simulink model "QAM16_PLL_Model"  (R2019a)
settings: Solver=FixedStepDiscrete  StartTime=0.0  StopTime=inf  FixedStep=1  RelTol=1e-3
undefined symbols (not defined in the file): DiscIntNeverNeededParam, i, jsin
libraries: commdigbbndam3 x3, commchan3 x1, commrandsrc3 x1
settings Model: Creator=vovan  LastModifiedBy=vovan
settings OptimizationCC: BlockReduction=off  DefaultParameterBehavior=Inlined  OptimizeBlockIOStorage=off  BufferReuse=off  GlobalBufferReuse=off  ExpressionFolding=off  PassReuseOutputArgsAs=Individual arguments  LocalBlockOutputs=off  OptimizeBlockOrder=speed  OptimizeDataStoreBuffers=off  BusAssignmentInplaceUpdate=off
settings DebuggingCC: ParameterTunabilityLossMsg=error
settings HardwareCC: TargetBitPerPointer=64  TargetBitPerSizeT=64  TargetBitPerPtrDiffT=64  TargetLongLongMode=on  TargetIntDivRoundTo=Zero  TargetEndianess=LittleEndian  TargetWordSize=64  TargetHWDeviceType=Generic->Custom  ProdEqTarget=off
settings SFSimCC: MATLABDynamicMemAlloc=off
settings RTWCC: SystemTargetFile=systemverilog_dpi_ert.tlc  TemplateMakefile=systemverilog_dpi_ert_default_tmf  Description=SystemVerilog DPI Component Generator  GenerateReport=on  IncludeHyperlinkInReport=on  LaunchReport=on  GenerateTraceInfo=on  GenerateTraceReport=on  GenerateTraceReportSl=on  GenerateTraceReportSf=on  GenerateTraceReportEml=on
settings CodeAppCC: ForceParamTrailComments=on  IgnoreCustomStorageClasses=off  MaxIdLength=256  OperatorAnnotations=on  SimulinkDataObjDesc=on  SFDataObjDesc=on  InsertBlockDesc=on
settings DPIERTTargetCC: TargetFcnLib=ansi_tfl_table_tmw.mat  GenFloatMathFcnCalls=NOT IN USE  TargetLangStandard=C89/C90 (ANSI)  CodeReplacementLibrary=None  UtilityFuncGeneration=Auto  MultiwordTypeDef=System defined  MultiwordLength=2048  DynamicStringBufferSize=256  GenerateFullHeader=on  InferredTypesCompatibility=off  GenerateSampleERTMain=off  GenerateTestInterfaces=off  ModelReferenceCompliant=on  ParMdlRefBuildCompliant=on  CompOptLevelCompliant=off  ConcurrentExecutionCompliant=off  IncludeMdlTerminateFcn=on  GeneratePreprocessorConditionals=Use local settings  CombineOutputUpdateFcns=off  CombineSignalStateStructs=on  GroupInternalDataByFunction=off  SuppressErrorStatus=off  IncludeFileDelimiter=Auto  ERTCustomFileBanners=on  SupportAbsoluteTime=on  LogVarNameModifier=rt_  MatFileLogging=off  MultiInstanceERTCode=on  CodeInterfacePackaging=Reusable function  PurelyIntegerCode=off  SupportNonFinite=on  SupportComplex=on  SupportContinuousTime=on  SupportNonInlinedSFcns=on  RemoveDisableFunc=off  RemoveResetFunc=on  SupportVariableSizeSignals=off  ParenthesesLevel=Nominal  CastingMode=Nominal  PreserveStateflowLocalDataDimensions=off  MATLABClassNameForMDSCustomization=Simulink.SoftwareTarget.TargetSpecificTriggerConfigurationBase  ModelStepFunctionPrototypeControlCompliant=on  CPPClassGenCompliant=off  AutosarCompliant=off  MDXCompliant=off  GRTInterface=off  GenerateAllocFcn=on  UseToolchainInfoCompliant=on  GenerateSharedConstants=on  CoderGroups=[]  AccessMethods=[]  LookupTableObjectStructAxisOrder=1,2,3,4,...  LUTObjectStructOrderExplicitValues=Size,Breakpoints,Table  LUTObjectStructOrderEvenSpacing=Size,Breakpoints,Table  ArrayLayout=Column-major  UnsupportedSFcnMsg=error  ERTHeaderFileRootName=$R$E  ERTSourceFileRootName=$R$E  ERTDataFileRootName=$R_data  GenerateASAP2=off  DSAsUniqueAccess=off  ExtMode=off  ExtModeTransport=0  ExtModeStaticAlloc=off  ExtModeStaticAllocSize=1000000  ExtModeTesting=off  ExtModeMexFile=ext_comm  ExtModeIntrfLevel=Level1  InlinedParameterPlacement=NonHierarchical  TargetOS=BareBoardExample  MultiInstanceErrorCode=Error  RootIOFormat=Part of model data structure  RTWCAPISignals=on  RTWCAPIParams=off  RTWCAPIStates=off  RTWCAPIRootIO=off  ERTSrcFileBannerTemplate=ert_code_template.cgt  ERTHdrFileBannerTemplate=ert_code_template.cgt  ERTDataSrcFileTemplate=ert_code_template.cgt  ERTDataHdrFileTemplate=ert_code_template.cgt  ERTCustomFileTemplate=example_file_process.tlc  EnableDataOwnership=off  SignalDisplayLevel=10  ParamTuneLevel=10  GlobalDataDefinition=Auto  DataDefinitionFile=global.c  GlobalDataReference=Auto  ERTFilePackagingFormat=Modular  RateTransitionBlockCode=Inline  DataReferenceFile=global.h  PreserveExpressionOrder=off  PreserveIfCondition=off  ConvertIfToSwitch=on  PreserveExternInFcnDecls=on  PreserveStaticInFcnDecls=on  SuppressUnreachableDefaultCases=on  EnableSignedLeftShifts=on  EnableSignedRightShifts=on  IndentStyle=K&R  IndentSize=2  NewlineStyle=Default  MaxLineWidth=80  EnableUserReplacementTypes=off  MaxIdInt64=MAX_int64_T  MinIdInt64=MIN_int64_T  MaxIdUint64=MAX_uint64_T  MaxIdInt32=MAX_int32_T  MinIdInt32=MIN_int32_T  MaxIdUint32=MAX_uint32_T  MaxIdInt16=MAX_int16_T  MinIdInt16=MIN_int16_T  MaxIdUint16=MAX_uint16_T  MaxIdInt8=MAX_int8_T  MinIdInt8=MIN_int8_T  MaxIdUint8=MAX_uint8_T  BooleanTrueId=true  BooleanFalseId=false  MemSecPackage=--- None ---  MemSecDataConstants=Default  MemSecDataIO=Default  MemSecDataInternal=Default  MemSecDataParameters=Default  MemSecFuncInitTerm=Default  MemSecFuncExecute=Default  MemSecFuncSharedUtil=Default  GroupConstants=Default  GroupRootInputs=Default  GroupRootOutputs=Default  GroupInternal=Default  GroupParameters=Default  GroupDataTransfer=Default  GroupSharedLocalDataStores=Default  GroupInstanceSpecificParameters=Default  GroupModelData=Default  DPICustomizeSystemVerilogCode=on  DPISystemVerilogTemplate=hdlverifier_dpitb_template.vgt  DPIGenerateTestBench=off  DPITestPointAccessFcnInterface=None  DPIFixedPointDataType=CompatibleCType  DPIPortConnection=Port list  DPICompositeDataType=Flattened

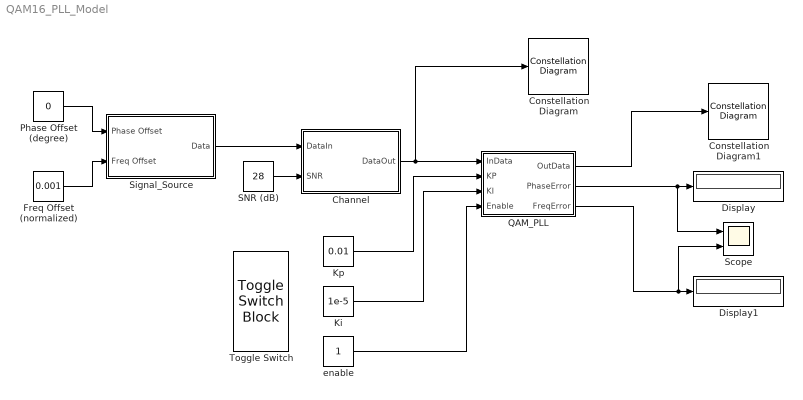
== system QAM16_PLL_Model ==
  Channel : Subsystem
  Constellation Diagram : ConstellationDiagram
  Constellation Diagram1 : ConstellationDiagram
  Display : Display
  Display1 : Display
  Freq Offset (normalized) : Constant  Value=0.001  SampleTime=1
  Ki : Constant  Value=1e-5  SampleTime=1
  Kp : Constant  Value=0.01  SampleTime=1
  Phase Offset (degree) : Constant  Value=0  SampleTime=1
  QAM_PLL : Subsystem
  SNR (dB) : Constant  Value=28  SampleTime=1
  Scope : Scope  NumInputPorts=2
  Signal_Source : Subsystem
  Toggle Switch : ToggleSwitchBlock
      settings: Values={{'Off', 'On'}, [0 1]}
  "enable " : Constant  OutDataTypeStr=boolean  SampleTime=1
  wires:
  Phase Offset (degree)/1 -> Signal_Source/1("Phase Offset ")
  Freq Offset (normalized)/1 -> Signal_Source/2(Freq Offset)
  Signal_Source/1(Data) -> Channel/1(DataIn)
  SNR (dB)/1 -> Channel/2(SNR)
  Channel/1(DataOut) -> QAM_PLL/1(InData), Constellation Diagram/1
  Kp/1 -> QAM_PLL/2(KP)
  Ki/1 -> QAM_PLL/3(KI)
  "enable "/1 -> QAM_PLL/4(Enable)
  QAM_PLL/1(OutData) -> Constellation Diagram1/1
  QAM_PLL/2(PhaseError) -> Scope/1, Display/1
  QAM_PLL/3(FreqError) -> Scope/2, Display1/1

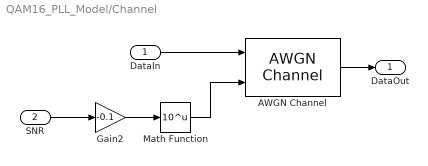
== system QAM16_PLL_Model/Channel ==
  DataIn : Inport
  SNR : Inport  Port=2
  AWGN Channel : commchan3/AWGN Channel  InputProcessing=Columns as channels (frame based)  seed=randseed  noiseMode=Variance from port  EbNodB=10  EsNodB=10  SNRdB=10  bitsPerSym=1  Ps=1  Tsym=1  variance=1
      settings: SourceProductName=Communications Toolbox
  Gain2 : Gain  Gain=-0.1
  Math Function : Math  Operator=10^u  SaturateOnIntegerOverflow=on
  DataOut : Outport
  wires:
  Math Function/1 -> AWGN Channel/2
  Gain2/1 -> Math Function/1
  DataIn/1 -> AWGN Channel/1
  AWGN Channel/1 -> DataOut/1
  SNR/1 -> Gain2/1

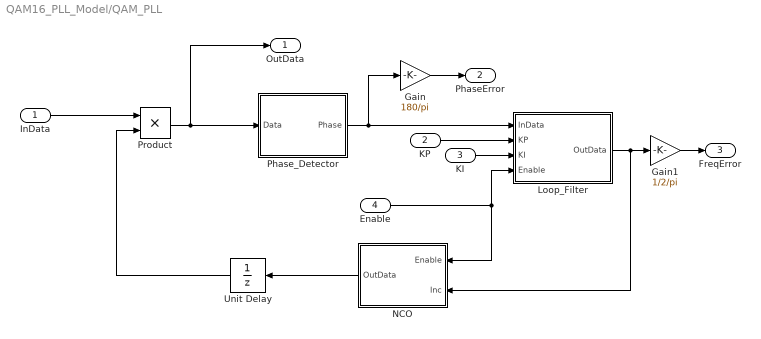
== system QAM16_PLL_Model/QAM_PLL ==
  InData : Inport
  KP : Inport  Port=2
  KI : Inport  Port=3
  Enable : Inport  Port=4
  Gain : Gain  Gain=180/pi
  Gain1 : Gain  Gain=1/2/pi
  Loop_Filter : Subsystem
  NCO : Subsystem
  Phase_Detector : Subsystem
  Product : Product
  Unit Delay : UnitDelay  SampleTime=-1  HasFrameUpgradeWarning=on
  OutData : Outport
  PhaseError : Outport  Port=2
  FreqError : Outport  Port=3
  wires:
  KP/1 -> Loop_Filter/2(KP)
  Enable/1 -> Loop_Filter/4(Enable), NCO/1(Enable)
  Phase_Detector/1(Phase) -> Gain/1, Loop_Filter/1(InData)
  Product/1 -> Phase_Detector/1(Data), OutData/1
  KI/1 -> Loop_Filter/3(KI)
  Loop_Filter/1(OutData) -> Gain1/1, NCO/2(Inc)
  NCO/1(OutData) -> Unit Delay/1
  Unit Delay/1 -> Product/2
  InData/1 -> Product/1
  Gain/1 -> PhaseError/1
  Gain1/1 -> FreqError/1

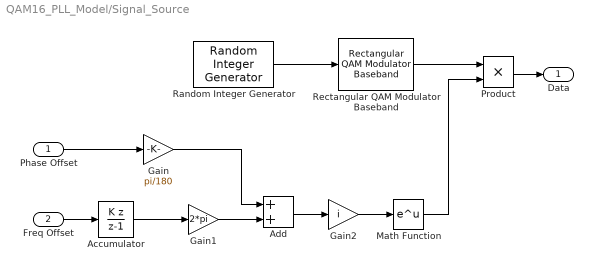
== system QAM16_PLL_Model/Signal_Source ==
  "Phase Offset " : Inport
  Freq Offset : Inport  Port=2
  Accumulator : DiscreteIntegrator  IntegratorMethod=Accumulation: Backward Euler  SampleTime=-1  ICPrevOutput=DiscIntNeverNeededParam  ICPrevScaledInput=DiscIntNeverNeededParam
  Add : Sum
  Gain : Gain  Gain=pi/180
  Gain1 : Gain  Gain=2*pi
  Gain2 : Gain  Gain=i
  Math Function : Math  SaturateOnIntegerOverflow=on
  Product : Product
  Random Integer Generator : commrandsrc3/Random Integer Generator  SetSize=16  SeedSource=Auto  Seed=0  SampleTime=1  SamplesPerFrame=1  OutputDataType=double  SimulateUsing=Interpreted execution
      settings: SourceProductName=Communications Toolbox
  Rectangular QAM Modulator Baseband : commdigbbndam3/Rectangular QAM Modulator Baseband  M=16  InType=Integer  Enc=Gray  Mapping=[0:15]  PowType=Average Power  MinDist=2  AvgPow=1  PeakPow=1  Ph=0  outDtype=double  outWordLen=16  outUDDataType=sfix(16)  outFracLenMode=Best precision  outFracLen=15  outDataTypeStr=double  outLastDataTypeStr=double
      settings: SourceProductName=Communications Toolbox
  Data : Outport
  wires:
  Gain/1 -> Add/1
  Rectangular QAM Modulator Baseband/1 -> Product/1
  Random Integer Generator/1 -> Rectangular QAM Modulator Baseband/1
  Freq Offset/1 -> Accumulator/1
  Gain1/1 -> Add/2
  Add/1 -> Gain2/1
  Gain2/1 -> Math Function/1
  Math Function/1 -> Product/2
  Accumulator/1 -> Gain1/1
  "Phase Offset "/1 -> Gain/1
  Product/1 -> Data/1

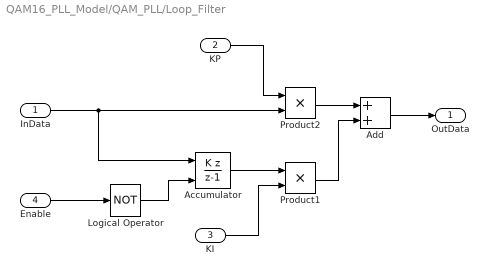
== system QAM16_PLL_Model/QAM_PLL/Loop_Filter ==
  InData : Inport
  KP : Inport  Port=2
  KI : Inport  Port=3
  Enable : Inport  Port=4  OutDataTypeStr=boolean
  Accumulator : DiscreteIntegrator  IntegratorMethod=Accumulation: Backward Euler  ExternalReset=level  SampleTime=-1  ICPrevOutput=DiscIntNeverNeededParam  ICPrevScaledInput=DiscIntNeverNeededParam
  Add : Sum
  Logical Operator : Logic  Operator=NOT  AllPortsSameDT=off  OutDataTypeStr=boolean
  Product1 : Product
  Product2 : Product
  OutData : Outport
  wires:
  InData/1 -> Accumulator/1, Product2/2
  Product2/1 -> Add/1
  Product1/1 -> Add/2
  KP/1 -> Product2/1
  Accumulator/1 -> Product1/1
  Add/1 -> OutData/1
  Enable/1 -> Logical Operator/1
  KI/1 -> Product1/2
  Logical Operator/1 -> Accumulator/2

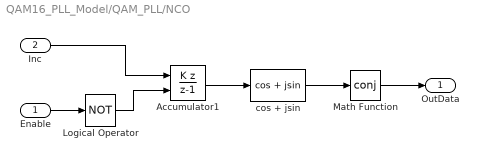
== system QAM16_PLL_Model/QAM_PLL/NCO ==
  Enable : Inport
  Inc : Inport  Port=2
  Accumulator1 : DiscreteIntegrator  IntegratorMethod=Accumulation: Backward Euler  ExternalReset=level  SampleTime=-1  ICPrevOutput=DiscIntNeverNeededParam  ICPrevScaledInput=DiscIntNeverNeededParam
  Logical Operator : Logic  Operator=NOT  AllPortsSameDT=off  OutDataTypeStr=boolean
  Math Function : Math  Operator=conj  SaturateOnIntegerOverflow=on
  cos + jsin : Trigonometry  Operator=cos + jsin
  OutData : Outport
  wires:
  Math Function/1 -> OutData/1
  Accumulator1/1 -> cos + jsin/1
  Enable/1 -> Logical Operator/1
  cos + jsin/1 -> Math Function/1
  Inc/1 -> Accumulator1/1
  Logical Operator/1 -> Accumulator1/2

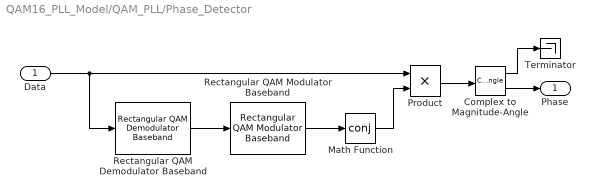
== system QAM16_PLL_Model/QAM_PLL/Phase_Detector ==
  Data : Inport
  Complex to Magnitude-Angle : ComplexToMagnitudeAngle
  Math Function : Math  Operator=conj  SaturateOnIntegerOverflow=on
  Product : Product
  Rectangular QAM Demodulator Baseband : commdigbbndam3/Rectangular QAM Demodulator Baseband  M=16  OutType=Integer  DecType=Hard decision  VarSource=Dialog  Variance=1  Dec=Gray  Mapping=[0:15]  PowType=Average Power  MinDist=2  AvgPow=1  PeakPow=1  Ph=0  outDtype1=Inherit via internal rule  outDtype2=Inherit via internal rule  derotateFactorWordLen=16  derotateFactorDataTypeStr=Inherit: Same word length as input  derotateFactorLastDataTypeStr=Inherit: Same word length as input  denormFactorWordLen=16  denormFactorDataTypeStr=Inherit: Same word length as input  denormFactorLastDataTypeStr=Inherit: Same word length as input  prodOutWordLen=32  prodOutOverflowMode=Wrap  prodOutRoundingMode=Floor  prodOutOvFlMode=off  prodOutOvFlModeLastStrValue=off  sumWordLen=32
      settings: SourceProductName=Communications Toolbox
  Rectangular QAM Modulator Baseband : commdigbbndam3/Rectangular QAM Modulator Baseband  M=16  InType=Integer  Enc=Gray  Mapping=[0:15]  PowType=Average Power  MinDist=2  AvgPow=1  PeakPow=1  Ph=0  outDtype=double  outWordLen=16  outUDDataType=sfix(16)  outFracLenMode=Best precision  outFracLen=15  outDataTypeStr=double  outLastDataTypeStr=double
      settings: SourceProductName=Communications Toolbox
  Terminator : Terminator
  Phase : Outport
  wires:
  Complex to Magnitude-Angle/1 -> Terminator/1
  Data/1 -> Product/1, Rectangular QAM Demodulator Baseband/1
  Rectangular QAM Modulator Baseband/1 -> Math Function/1
  Rectangular QAM Demodulator Baseband/1 -> Rectangular QAM Modulator Baseband/1
  Complex to Magnitude-Angle/2 -> Phase/1
  Product/1 -> Complex to Magnitude-Angle/1
  Math Function/1 -> Product/2
